simulink model "Embedded_Ex3"  (R2022a)
settings: Solver=FixedStepDiscrete  StartTime=0.0  StopTime=10.0  FixedStep=1  RelTol=1e-3  EnableMultiTasking=on
settings Model: ExtModeTrigDuration=2  Creator=aminsaveh  LastModifiedBy=aminsaveh
settings OptimizationCC: EnhancedBackFolding=on  PassReuseOutputArgsAs=Individual arguments  ZeroExternalMemoryAtStartup=off  ZeroInternalMemoryAtStartup=off  MaxStackSize=64  OptimizeBlockOrder=speed  DifferentSizesBufferReuse=on  OptimizationCustomize=off  EfficientTunableParamExpr=on
settings DebuggingCC: ParameterTunabilityLossMsg=error
settings HardwareCC: ProdBitPerInt=16  ProdBitPerPointer=16  ProdBitPerSizeT=16  ProdBitPerPtrDiffT=16  ProdLargestAtomicFloat=None  ProdWordSize=8  ProdHWDeviceType=Atmel->AVR
settings SFSimCC: MATLABDynamicMemAlloc=off
settings RTWCC: SystemTargetFile=ert.tlc  HardwareBoard=Arduino Uno  GenCodeOnly=on  TemplateMakefile=ert_default_tmf  Toolchain=Arduino AVR  BuildConfiguration=Faster Runs
settings CodeAppCC: ForceParamTrailComments=on  IgnoreCustomStorageClasses=off  OperatorAnnotations=on  SimulinkDataObjDesc=on  SFDataObjDesc=on  InsertBlockDesc=on
settings ERTTargetCC: TargetLangStandard=C99 (ISO)  SupportContinuousTime=on  SupportVariableSizeSignals=on  ExtModeTransport=3  ExtModeStaticAlloc=on  ExtModeStaticAllocSize=250  ExtModeMexFile=ext_xcp  ExtModeIntrfLevel=Level2 - Open

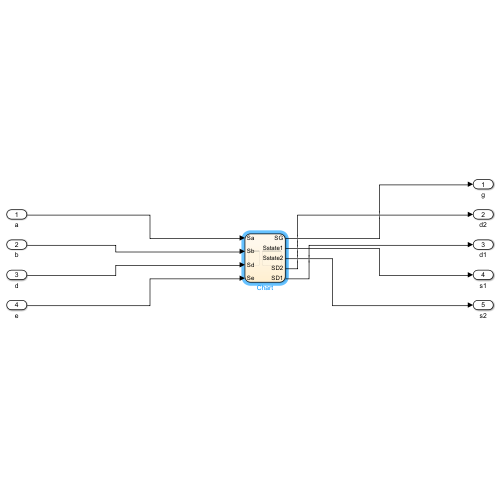
[thumbnail: Simulink's stored preview of the top-level diagram]
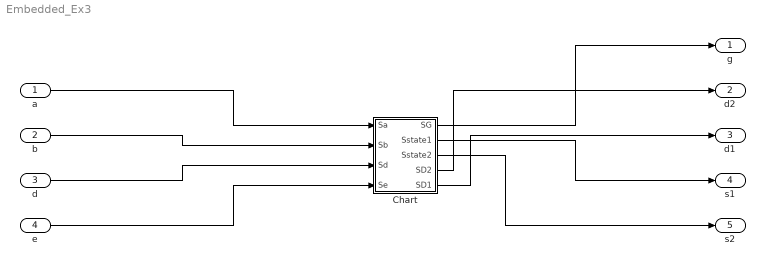
== system Embedded_Ex3 ==
  a : Inport
  b : Inport  Port=2
  d : Inport  Port=3
  e : Inport  Port=4
  Chart : Stateflow chart  TreatAsAtomicUnit=on
  g : Outport
  d2 : Outport  Port=2
  d1 : Outport  Port=3
  s1 : Outport  Port=4
  s2 : Outport  Port=5
  wires:
  a/1 -> Chart/1(Sa)
  b/1 -> Chart/2(Sb)
  d/1 -> Chart/3(Sd)
  e/1 -> Chart/4(Se)
  Chart/1(SG) -> g/1
  Chart/2(Sstate1) -> s1/1
  Chart/3(Sstate2) -> s2/1
  Chart/5(SD1) -> d1/1
  Chart/4(SD2) -> d2/1

== stateflow chart Embedded_Ex3/Chart ==
  settings: sampleTime=1
  state B [parallel]
    settings: executionOrder=2
    state state1
    state state2
    (default) -> state1 : {Sstate1=true;}
    state1 -> state2 : [c==true]{Sstate1=false;Sstate2=true;}
    state2 -> state1 : [Sb == true && in(C.D.D2)]{Sstate1=true;Sstate2=false;}
  state C [parallel]
    settings: executionOrder=1
    state D
      state D1
      state D2
      (default) -> D1 : {SD1=true;SG=false;}
      D1 -> D2 : [Se==true]{SD2 = true;SD1= false;c = false;}
      D2 -> D2 : [Se==true]{SD2= true;}
    state G
    G -> D : [Sa==true]{c = true;SG=false;}
    (default) -> G : {SG=true;}
    D -> G : [Sd==true]{SD2=false;SG=true;}
  data: c local size=1 =false; SG output =false; Sstate1 output =false; Sstate2 output =false; Sa input boolean; Sb input boolean; Sd input boolean; Se input boolean; SD2 output =false; SD1 output =false
